simulink model "SimulationANTSMC"  (R2020b)
(part 1 of 18)
settings: Solver=ode3  StartTime=0.0  StopTime=100  FixedStep=0.001  RelTol=1e-6  EnableMultiTasking=on
model workspace (MAT data in the model file):
  time = 1
values from neighbouring files (symbols this model uses):
  beta = 2*x(3)/(1+x(3))    [GA_init.m]
  epstar = x(9)    [GA_init.m]
  g0 = x(5)    [GA_init.m]
  g1 = x(6)    [GA_init.m]
  g2 = x(7)    [GA_init.m]
  g3 = x(8)    [GA_init.m]
  gamma = x(3)    [GA_init.m]
  kappa = x(11)    [GA_init.m]
  landa = x(1)    [GA_init.m]
  nu = x(2)    [GA_init.m]
  vu = x(4)    [GA_init.m]

== system SimulationANTSMC ==
  Constant : Constant  Value=[0.00000000001*ones(6,1);zeros(6,1)]
  Control signal : Scope
  Disturbance : Scope
  Joint Trajectory : Subsystem
  Psi : Scope
  S : Scope
  Subsystem : Subsystem
  To Workspace : ToWorkspace  VariableName=error  SampleTime=-1
  To Workspace1 : ToWorkspace  VariableName=control_signal  SampleTime=-1
  Uas : Scope
  error : Scope
  thetadot : Scope
  track : Scope  NumInputPorts=2
  wires:
  Joint Trajectory/1(thetad) -> track/1, Subsystem/1(Xd)
  Subsystem/2(Error) -> error/1, To Workspace/1
  Subsystem/5(Control Signal) -> Control signal/1, To Workspace1/1
  Subsystem/1(theta) -> track/2
  Subsystem/3(thetadot) -> thetadot/1
  Subsystem/4(S) -> S/1
  Subsystem/6(Disturbance) -> Disturbance/1
  Constant/1 -> Subsystem/2(Initial)
  Subsystem/7(Us) -> Uas/1
  Subsystem/8(Psi1) -> Psi/1

== system SimulationANTSMC/Joint Trajectory ==
  Clock1 : Clock
  Mux : Mux  Inputs=6
  Mux1 : Mux  Commented=on  Inputs=6
  Sine Wave Function : Sin  TimeSource=Use external signal  Frequency=0.1*2*pi  SampleTime=0
  Sine Wave Function1 : Sin  TimeSource=Use external signal  Frequency=0.1*2*pi  SampleTime=0
  Sine Wave Function2 : Sin  TimeSource=Use external signal  Frequency=0.1*2*pi  SampleTime=0
  Sine Wave Function3 : Sin  TimeSource=Use external signal  Amplitude=-1  Frequency=0.1*2*pi  SampleTime=0
  Sine Wave Function4 : Sin  TimeSource=Use external signal  Amplitude=-1  Frequency=0.1*2*pi  SampleTime=0
  Sine Wave Function5 : Sin  TimeSource=Use external signal  Amplitude=-1  Frequency=0.1*2*pi  SampleTime=0
  Step : Step  Commented=on  Time=0  After=-5  SampleTime=0
  Step1 : Step  Commented=on  Time=0  After=-5  SampleTime=0
  Step2 : Step  Commented=on  Time=0  After=-1  SampleTime=0
  Step3 : Step  Commented=on  Time=0  After=5  SampleTime=0
  Step4 : Step  Commented=on  Time=0  After=5  SampleTime=0
  Step5 : Step  Commented=on  Time=0  After=5  SampleTime=0
  thetad : Outport
  wires:
  Clock1/1 -> Sine Wave Function5/1, Sine Wave Function4/1, Sine Wave Function1/1, Sine Wave Function/1, Sine Wave Function2/1, Sine Wave Function3/1
  Step3/1 -> Mux1/4
  Step4/1 -> Mux1/5
  Step5/1 -> Mux1/6
  Step2/1 -> Mux1/1
  Step1/1 -> Mux1/2
  Step/1 -> Mux1/3
  Mux/1 -> thetad/1
  Sine Wave Function5/1 -> Mux/1
  Sine Wave Function4/1 -> Mux/2
  Sine Wave Function3/1 -> Mux/3
  Sine Wave Function2/1 -> Mux/4
  Sine Wave Function1/1 -> Mux/5
  Sine Wave Function/1 -> Mux/6

== system SimulationANTSMC/Subsystem ==
  Xd : Inport
  Initial : Inport  Port=2
  Clock : Clock
  Constant1 : Constant  Value=landa
  Derivative{,1..3} (4 alike) : Derivative
  Design Parameters : Constant  Value=[g0,g1,g2,g3,gamma,beta]'
  Integrator : Integrator  InitialConditionSource=external  InitialCondition=[1*ones(6,1);ones(6,1)]  UpperSaturationLimit=10000  LowerSaturationLimit=-10000  AbsoluteTolerance=-1  ZeroCross=off
  Integrator1 : Integrator  InitialCondition=[0*ones(6,1)]  UpperSaturationLimit=1000  LowerSaturationLimit=-1000  AbsoluteTolerance=-1
  Mux : Mux  Inputs=6
  S manifold : MATLAB Function  TreatAsAtomicUnit=on
  Signal Specification{,1..3} (4 alike) : SignalSpecification  Dimensions=6
  Sum : Sum  Inputs=-|+
  Sum1 : Sum  Inputs=+|+
  System Dynamics : MATLAB Function  TreatAsAtomicUnit=on
  Theta : Subsystem
  To Workspace2 : ToWorkspace  VariableName=time  SampleTime=-1
  U : MATLAB Function  TreatAsAtomicUnit=on
  Uas : Subsystem
  Ueq : MATLAB Function  TreatAsAtomicUnit=on
  theta : Outport
  Error : Outport  Port=2
  thetadot : Outport  Port=3
  S : Outport  Port=4
  Control Signal : Outport  Port=5
  Disturbance : Outport  Port=6
  Us : Outport  Port=7
  Psi1 : Outport  Port=8
  wires:
  Sum1/1 -> Integrator1/1  "S"
  Constant1/1 -> Ueq/5(landa)
  Signal Specification1/1 -> Ueq/9(thetadot), U/4(thetadot), System Dynamics/2(thetadot)
  Clock/1 -> System Dynamics/4(t), To Workspace2/1
  System Dynamics/2(y) -> Integrator/1
  Design Parameters/1 -> S manifold/1(despar), Ueq/4(despar)
  Integrator/1 -> Theta/1(In1)
  Derivative/1 -> Ueq/7(edot), Derivative3/1, S manifold/3(edot)
  Theta/2(thetadot) -> Signal Specification1/1, thetadot/1
  Theta/1(theta) -> Signal Specification/1
  Derivative2/1 -> Ueq/1(xddd)
  Derivative1/1 -> Derivative2/1
  Sum/1 -> Ueq/3(e), Error/1, S manifold/2(e), Derivative/1  "Error"
  Ueq/1(y) -> Signal Specification2/1
  Signal Specification/1 -> theta/1, Sum/2, Ueq/8(theta), U/3(theta), System Dynamics/3(theta)
  Mux/1 -> Sum1/1, Ueq/6(part)
  Xd/1 -> Derivative1/1, Sum/1
  System Dynamics/1(disturbance) -> Disturbance/1
  S manifold/5(z5) -> Mux/5
  S manifold/1(z1) -> Mux/1
  S manifold/3(z3) -> Mux/3
  S manifold/4(z4) -> Mux/4
  S manifold/6(z6) -> Mux/6
  S manifold/2(z2) -> Mux/2
  Signal Specification2/1 -> U/1(Ueq)
  U/1(u) -> Control Signal/1, System Dynamics/1(u)
  Initial/1 -> Integrator/2
  Uas/1(Uas) -> U/2(Uas), Us/1
  Uas/2(Psi) -> Psi1/1
  Derivative3/1 -> Sum1/2
  Integrator1/1 -> Signal Specification3/1, Ueq/2(S)
  Signal Specification3/1 -> Uas/1(S), S/1

== system SimulationANTSMC/Subsystem/Theta ==
  In1 : Inport
  Bus Creator2 : BusCreator  Commented=on  Inputs=6
  Bus Creator3 : BusCreator  Commented=on  Inputs=6
  Subsystem : Subsystem  Commented=on
  Subsystem1 : Subsystem  Commented=on
  Subsystem2 : Subsystem  Commented=on
  Subsystem3 : Subsystem  Commented=on
  Subsystem4 : Subsystem  Commented=on
  Subsystem5 : Subsystem  Commented=on
  Subsystem6 : Subsystem  Commented=on
  Terminator : Terminator
  Theta : Subsystem
  theta : Outport
  thetadot : Outport  Port=2
  wires:
  Subsystem/3(Out3) -> Subsystem3/1(In1)  "theta3"
  Subsystem/6(Out6) -> Subsystem6/1(In1)  "theta6"
  Subsystem/4(Out4) -> Subsystem4/1(In1)  "theta4"
  Subsystem/11(Out11) -> Bus Creator3/5
  Subsystem/1(Out1) -> Subsystem1/1(In1)  "theta1"
  Subsystem/9(Out9) -> Bus Creator3/3
  Subsystem/12(Out12) -> Bus Creator3/6
  Subsystem/5(Out5) -> Subsystem5/1(In1)  "theta5"
  Subsystem/10(Out10) -> Bus Creator3/4
  Subsystem/8(Out8) -> Bus Creator3/2
  Subsystem/2(Out2) -> Subsystem2/1(In1)  "theta2"
  Subsystem/7(Out7) -> Bus Creator3/1
  Subsystem2/1(Out1) -> Bus Creator2/2
  Subsystem1/1(Out1) -> Bus Creator2/1
  Subsystem6/1(Out1) -> Bus Creator2/6
  Subsystem3/1(Out1) -> Bus Creator2/3
  Subsystem4/1(Out1) -> Bus Creator2/4
  Subsystem5/1(Out1) -> Bus Creator2/5
  In1/1 -> Theta/1(In1)
  Theta/1(Theta Degree) -> Terminator/1
  Theta/2(thetadot) -> thetadot/1
  Theta/3(Theta Radian) -> theta/1

== system SimulationANTSMC/Subsystem/Uas ==
  S : Inport
  Add2 : Sum
  Constant1 : Constant  Value=epstar
  Constant2 : Constant  Value=kappa
  Constant3 : Constant  Value=nu
  Constant4 : Constant  Value=vu
  Integrator2 : Integrator
  MATLAB Function : MATLAB Function  TreatAsAtomicUnit=on
  MATLAB Function1 : MATLAB Function  TreatAsAtomicUnit=on
  Product : Product
  Signal Specification : SignalSpecification  Dimensions=6
  Uas : Outport
  Psi : Outport  Port=2
  wires:
  Integrator2/1 -> Add2/2, Psi/1  "Psi"
  Add2/1 -> Product/2  "S"
  Constant2/1 -> MATLAB Function1/2(kappa)
  Constant3/1 -> Add2/1
  Product/1 -> Uas/1
  Constant1/1 -> MATLAB Function/2(epstar)
  Constant4/1 -> MATLAB Function1/3(vu)
  MATLAB Function/1(sat) -> Product/1
  MATLAB Function1/1(psi_dot) -> Signal Specification/1
  S/1 -> MATLAB Function/1(s), MATLAB Function1/1(s)
  Signal Specification/1 -> Integrator2/1

== system SimulationANTSMC/Subsystem/Theta/Subsystem ==
  In1 : Inport
  Demux3 : Demux  Outputs=12
  Out1 : Outport
  Out2 : Outport  Port=2
  Out3 : Outport  Port=3
  Out4 : Outport  Port=4
  Out5 : Outport  Port=5
  Out6 : Outport  Port=6
  Out7 : Outport  Port=7
  Out8 : Outport  Port=8
  Out9 : Outport  Port=9
  Out10 : Outport  Port=10
  Out11 : Outport  Port=11
  Out12 : Outport  Port=12
  wires:
  Demux3/1 -> Out1/1
  Demux3/9 -> Out9/1
  Demux3/10 -> Out10/1
  Demux3/7 -> Out7/1
  In1/1 -> Demux3/1
  Demux3/8 -> Out8/1
  Demux3/11 -> Out11/1
  Demux3/5 -> Out5/1
  Demux3/3 -> Out3/1
  Demux3/2 -> Out2/1
  Demux3/4 -> Out4/1
  Demux3/6 -> Out6/1
  Demux3/12 -> Out12/1

== system SimulationANTSMC/Subsystem/Theta/Subsystem1 ==
  In1 : Inport
  Constant2 : Constant  Value=360
  Gain : Gain  Gain=pi/180
  Math Function : Math  Operator=rem  SignedPower=on
  Out1 : Outport
  wires:
  Math Function/1 -> Out1/1
  In1/1 -> Gain/1
  Constant2/1 -> Math Function/2
  Gain/1 -> Math Function/1

== system SimulationANTSMC/Subsystem/Theta/Subsystem2 ==
  In1 : Inport
  Constant2 : Constant  Value=360
  Gain : Gain  Gain=pi/180
  Math Function : Math  Operator=rem  SignedPower=on
  Out1 : Outport
  wires:
  Math Function/1 -> Out1/1
  In1/1 -> Gain/1
  Constant2/1 -> Math Function/2
  Gain/1 -> Math Function/1

== system SimulationANTSMC/Subsystem/Theta/Subsystem3 ==
  In1 : Inport
  Constant2 : Constant  Value=360
  Gain : Gain  Gain=pi/180
  Math Function : Math  Operator=rem  SignedPower=on
  Out1 : Outport
  wires:
  Math Function/1 -> Out1/1
  In1/1 -> Gain/1
  Constant2/1 -> Math Function/2
  Gain/1 -> Math Function/1

== system SimulationANTSMC/Subsystem/Theta/Subsystem4 ==
  In1 : Inport
  Constant2 : Constant  Value=360
  Gain : Gain  Gain=pi/180
  Math Function : Math  Operator=rem  SignedPower=on
  Out1 : Outport
  wires:
  Math Function/1 -> Out1/1
  In1/1 -> Gain/1
  Constant2/1 -> Math Function/2
  Gain/1 -> Math Function/1
(part 1 of 6)
settings Model: Creator=CAST ta 1400  LastModifiedBy=Hirsa
settings DataIOCC: ReturnWorkspaceOutputs=off
settings OptimizationCC: LifeSpan=inf
settings DebuggingCC: SFUnexpectedBacktrackingDiag=warning  SFNoUnconditionalDefaultTransitionDiag=warning  ArithmeticOperatorsInVariantConditions=warning
settings SFSimCC: SimUseLocalCustomCode=off  CustomCodeUndefinedFunction=UseInterfaceOnly
settings RTWCC: RTWUseLocalCustomCode=off
settings CodeAppCC: StateflowObjectComments=on
settings GRTTargetCC: TargetLangStandard=C89/C90 (ANSI)
settings ConfigComp: CovMetricSettings=dw  CovSaveCumulativeToWorkspaceVar=on  CovSaveSingleToWorkspaceVar=on  CovExternalEMLEnable=off

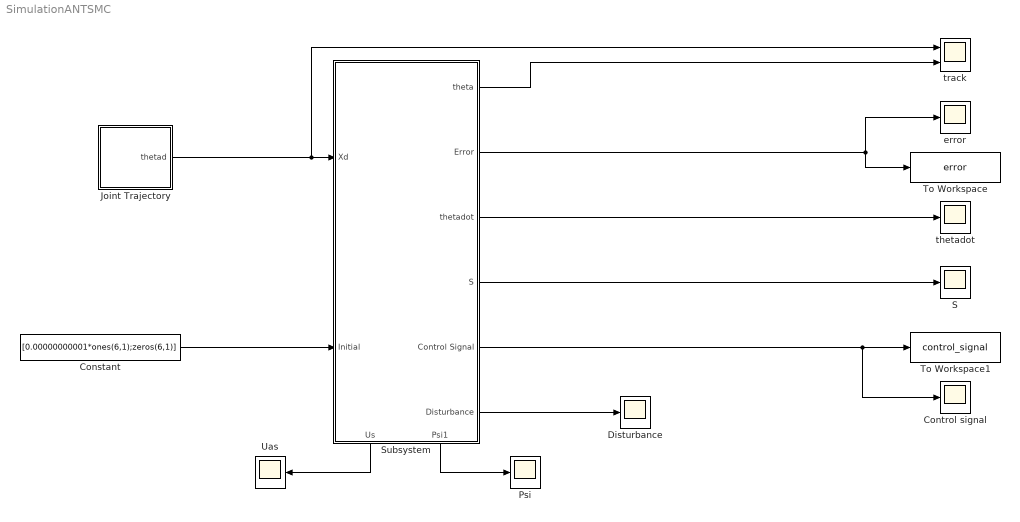
== system SimulationANTSMC ==
  Constant : Constant  Value=[0.00000000001*ones(6,1);zeros(6,1)]
  Control signal : Scope
  Disturbance : Scope
  Joint Trajectory : Subsystem
  Psi : Scope
  S : Scope
  Subsystem : Subsystem
      settings: PortSchema="{\"entries\":[{\"content\":{\"sides\":[{\"content\":{\"connectorIds\":[\"In1\",\"In2\"]},\"type\":\"ConnectorPlacement.EquallySpacedRectSide\",\"uuid\":\"6a081601-8c1c-4b92-8876-618e6a79f348\"},{\"content\":{\"connectorIds\":[\"Out1\",\"Out2\",\"Out3\",\"Out4\",\"Out5\",\"Out6\"],\"side\":\"RIGHT\"},\"type\":\"ConnectorPlacement.EquallySpacedRectSide\",\"uuid\":\"d972793b-0164-4612-badd-e3b053e392fc\"},{\"content\":{\"connectorIds\":[],\"side\":\"TOP\"},\"type\":\"ConnectorPlacement.EquallySpacedRectSide\",\"uuid\":\"780efbe4-9119-4fa0-8e03-d919fd60940e\"},{\"content\":{\"connectorIds\":[\"Out7\",\"Out8\"],\"side\":\"BOTTOM\"},\"type\":\"ConnectorPlacement.EquallySpacedRectSide\",\"uuid\":\"2e229f1a-e48e-496e-b525-7ed2e3990976\"},{\"content\":{\"connectorIds\":[],\"side\":\"HIDDEN\"},\"type\":\"ConnectorPlacement.EquallySpacedRectSide\",\"uuid\":\"e6c47cfa-e173-45ed-863d-94438e578280\"}]},\"type\":\"ConnectorPlacement.EquallySpacedConnector\",\"uuid\":\"71e70820-15e2-4153-83ec-01219cd454a2\"}],\"packageUris\":[\"http://schema.mathworks.com/mf0/Connector/R2020b\"],\"version\":\"1.0\"}"
  To Workspace : ToWorkspace  VariableName=error  SampleTime=-1
  To Workspace1 : ToWorkspace  VariableName=control_signal  SampleTime=-1
  Uas : Scope
  error : Scope
  thetadot : Scope
  track : Scope  NumInputPorts=2
  wires:
  Joint Trajectory/1(thetad) -> track/1, Subsystem/1(Xd)
  Subsystem/2(Error) -> error/1, To Workspace/1
  Subsystem/5(Control Signal) -> Control signal/1, To Workspace1/1
  Subsystem/1(theta) -> track/2
  Subsystem/3(thetadot) -> thetadot/1
  Subsystem/4(S) -> S/1
  Subsystem/6(Disturbance) -> Disturbance/1
  Constant/1 -> Subsystem/2(Initial)
  Subsystem/7(Us) -> Uas/1
  Subsystem/8(Psi1) -> Psi/1

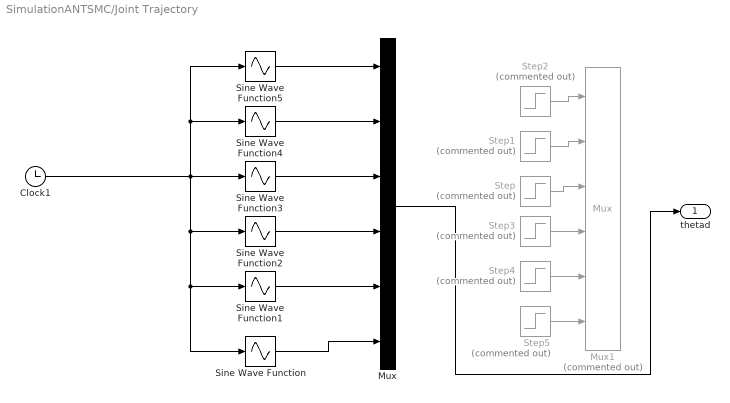
== system SimulationANTSMC/Joint Trajectory ==
  Clock1 : Clock
  Mux : Mux  Inputs=6
  Mux1 : Mux  Commented=on  Inputs=6
  Sine Wave Function : Sin  TimeSource=Use external signal  Frequency=0.1*2*pi  SampleTime=0
  Sine Wave Function1 : Sin  TimeSource=Use external signal  Frequency=0.1*2*pi  SampleTime=0
  Sine Wave Function2 : Sin  TimeSource=Use external signal  Frequency=0.1*2*pi  SampleTime=0
  Sine Wave Function3 : Sin  TimeSource=Use external signal  Amplitude=-1  Frequency=0.1*2*pi  SampleTime=0
  Sine Wave Function4 : Sin  TimeSource=Use external signal  Amplitude=-1  Frequency=0.1*2*pi  SampleTime=0
  Sine Wave Function5 : Sin  TimeSource=Use external signal  Amplitude=-1  Frequency=0.1*2*pi  SampleTime=0
  Step : Step  Commented=on  Time=0  After=-5  SampleTime=0
  Step1 : Step  Commented=on  Time=0  After=-5  SampleTime=0
  Step2 : Step  Commented=on  Time=0  After=-1  SampleTime=0
  Step3 : Step  Commented=on  Time=0  After=5  SampleTime=0
  Step4 : Step  Commented=on  Time=0  After=5  SampleTime=0
  Step5 : Step  Commented=on  Time=0  After=5  SampleTime=0
  thetad : Outport
  wires:
  Clock1/1 -> Sine Wave Function5/1, Sine Wave Function4/1, Sine Wave Function1/1, Sine Wave Function/1, Sine Wave Function2/1, Sine Wave Function3/1
  Step3/1 -> Mux1/4
  Step4/1 -> Mux1/5
  Step5/1 -> Mux1/6
  Step2/1 -> Mux1/1
  Step1/1 -> Mux1/2
  Step/1 -> Mux1/3
  Mux/1 -> thetad/1
  Sine Wave Function5/1 -> Mux/1
  Sine Wave Function4/1 -> Mux/2
  Sine Wave Function3/1 -> Mux/3
  Sine Wave Function2/1 -> Mux/4
  Sine Wave Function1/1 -> Mux/5
  Sine Wave Function/1 -> Mux/6

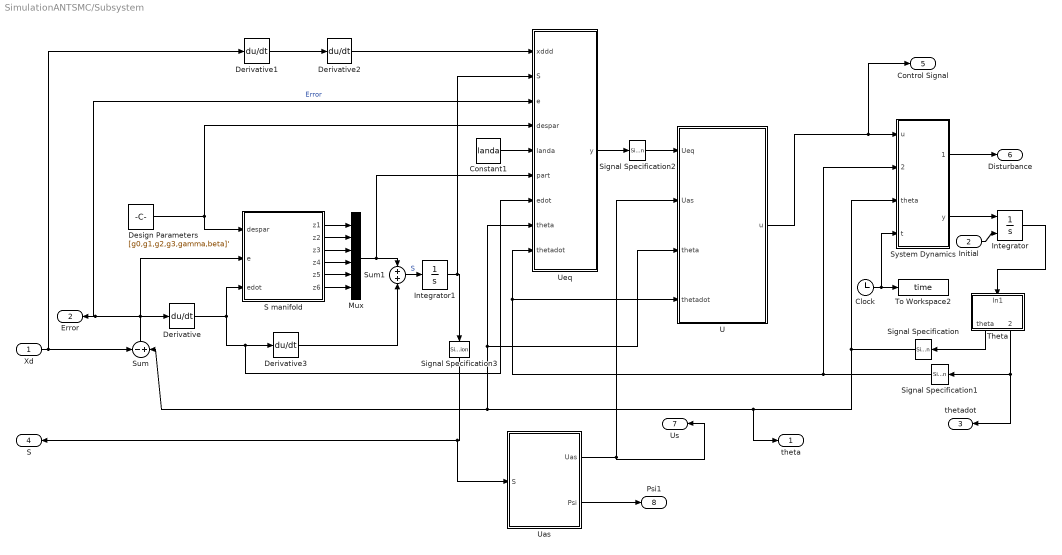
== system SimulationANTSMC/Subsystem ==
  Xd : Inport
  Initial : Inport  Port=2
  Clock : Clock
  Constant1 : Constant  Value=landa
  Derivative{,1..3} (4 alike) : Derivative
  Design Parameters : Constant  Value=[g0,g1,g2,g3,gamma,beta]'
  Integrator : Integrator  InitialConditionSource=external  InitialCondition=[1*ones(6,1);ones(6,1)]  UpperSaturationLimit=10000  LowerSaturationLimit=-10000  AbsoluteTolerance=-1  ZeroCross=off
  Integrator1 : Integrator  InitialCondition=[0*ones(6,1)]  UpperSaturationLimit=1000  LowerSaturationLimit=-1000  AbsoluteTolerance=-1
  Mux : Mux  Inputs=6
  S manifold : MATLAB Function  TreatAsAtomicUnit=on
  Signal Specification{,1..3} (4 alike) : SignalSpecification  Dimensions=6
  Sum : Sum  Inputs=-|+
  Sum1 : Sum  Inputs=+|+
  System Dynamics : MATLAB Function  TreatAsAtomicUnit=on
  Theta : Subsystem
  To Workspace2 : ToWorkspace  VariableName=time  SampleTime=-1
  U : MATLAB Function  TreatAsAtomicUnit=on
  Uas : Subsystem
  Ueq : MATLAB Function  TreatAsAtomicUnit=on
  theta : Outport
  Error : Outport  Port=2
  thetadot : Outport  Port=3
  S : Outport  Port=4
  Control Signal : Outport  Port=5
  Disturbance : Outport  Port=6
  Us : Outport  Port=7
  Psi1 : Outport  Port=8
  wires:
  Sum1/1 -> Integrator1/1  "S"
  Constant1/1 -> Ueq/5(landa)
  Signal Specification1/1 -> Ueq/9(thetadot), U/4(thetadot), System Dynamics/2(thetadot)
  Clock/1 -> System Dynamics/4(t), To Workspace2/1
  System Dynamics/2(y) -> Integrator/1
  Design Parameters/1 -> S manifold/1(despar), Ueq/4(despar)
  Integrator/1 -> Theta/1(In1)
  Derivative/1 -> Ueq/7(edot), Derivative3/1, S manifold/3(edot)
  Theta/2(thetadot) -> Signal Specification1/1, thetadot/1
  Theta/1(theta) -> Signal Specification/1
  Derivative2/1 -> Ueq/1(xddd)
  Derivative1/1 -> Derivative2/1
  Sum/1 -> Ueq/3(e), Error/1, S manifold/2(e), Derivative/1  "Error"
  Ueq/1(y) -> Signal Specification2/1
  Signal Specification/1 -> theta/1, Sum/2, Ueq/8(theta), U/3(theta), System Dynamics/3(theta)
  Mux/1 -> Sum1/1, Ueq/6(part)
  Xd/1 -> Derivative1/1, Sum/1
  System Dynamics/1(disturbance) -> Disturbance/1
  S manifold/5(z5) -> Mux/5
  S manifold/1(z1) -> Mux/1
  S manifold/3(z3) -> Mux/3
  S manifold/4(z4) -> Mux/4
  S manifold/6(z6) -> Mux/6
  S manifold/2(z2) -> Mux/2
  Signal Specification2/1 -> U/1(Ueq)
  U/1(u) -> Control Signal/1, System Dynamics/1(u)
  Initial/1 -> Integrator/2
  Uas/1(Uas) -> U/2(Uas), Us/1
  Uas/2(Psi) -> Psi1/1
  Derivative3/1 -> Sum1/2
  Integrator1/1 -> Signal Specification3/1, Ueq/2(S)
  Signal Specification3/1 -> Uas/1(S), S/1

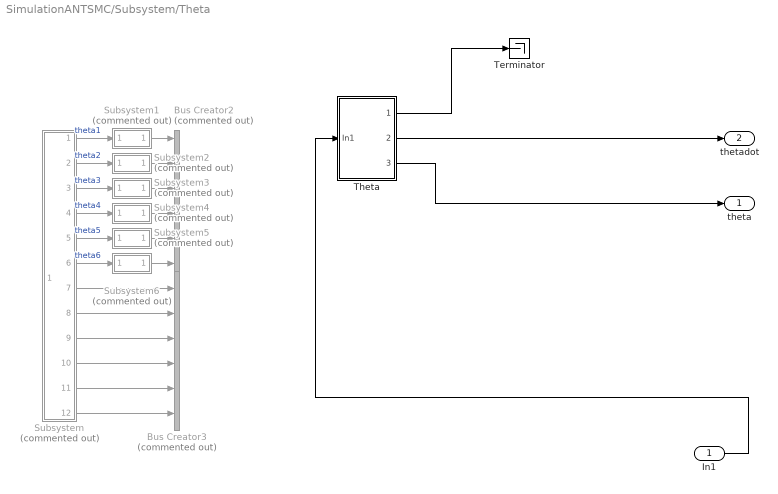
== system SimulationANTSMC/Subsystem/Theta ==
  In1 : Inport
  Bus Creator2 : BusCreator  Commented=on  Inputs=6
  Bus Creator3 : BusCreator  Commented=on  Inputs=6
  Subsystem : Subsystem  Commented=on
  Subsystem1 : Subsystem  Commented=on
  Subsystem2 : Subsystem  Commented=on
  Subsystem3 : Subsystem  Commented=on
  Subsystem4 : Subsystem  Commented=on
  Subsystem5 : Subsystem  Commented=on
  Subsystem6 : Subsystem  Commented=on
  Terminator : Terminator
  Theta : Subsystem
  theta : Outport
  thetadot : Outport  Port=2
  wires:
  Subsystem/3(Out3) -> Subsystem3/1(In1)  "theta3"
  Subsystem/6(Out6) -> Subsystem6/1(In1)  "theta6"
  Subsystem/4(Out4) -> Subsystem4/1(In1)  "theta4"
  Subsystem/11(Out11) -> Bus Creator3/5
  Subsystem/1(Out1) -> Subsystem1/1(In1)  "theta1"
  Subsystem/9(Out9) -> Bus Creator3/3
  Subsystem/12(Out12) -> Bus Creator3/6
  Subsystem/5(Out5) -> Subsystem5/1(In1)  "theta5"
  Subsystem/10(Out10) -> Bus Creator3/4
  Subsystem/8(Out8) -> Bus Creator3/2
  Subsystem/2(Out2) -> Subsystem2/1(In1)  "theta2"
  Subsystem/7(Out7) -> Bus Creator3/1
  Subsystem2/1(Out1) -> Bus Creator2/2
  Subsystem1/1(Out1) -> Bus Creator2/1
  Subsystem6/1(Out1) -> Bus Creator2/6
  Subsystem3/1(Out1) -> Bus Creator2/3
  Subsystem4/1(Out1) -> Bus Creator2/4
  Subsystem5/1(Out1) -> Bus Creator2/5
  In1/1 -> Theta/1(In1)
  Theta/1(Theta Degree) -> Terminator/1
  Theta/2(thetadot) -> thetadot/1
  Theta/3(Theta Radian) -> theta/1

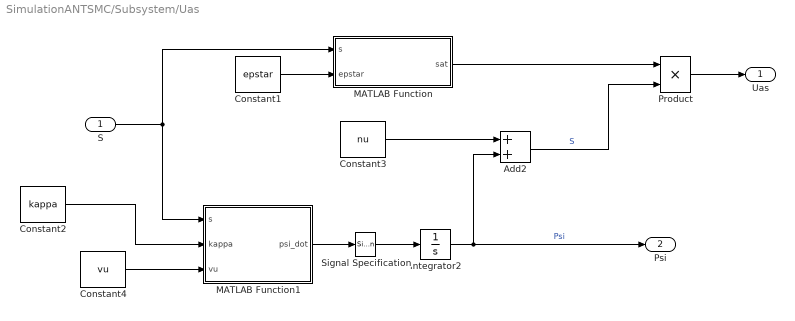
== system SimulationANTSMC/Subsystem/Uas ==
  S : Inport
  Add2 : Sum
  Constant1 : Constant  Value=epstar
  Constant2 : Constant  Value=kappa
  Constant3 : Constant  Value=nu
  Constant4 : Constant  Value=vu
  Integrator2 : Integrator
  MATLAB Function : MATLAB Function  TreatAsAtomicUnit=on
  MATLAB Function1 : MATLAB Function  TreatAsAtomicUnit=on
  Product : Product
  Signal Specification : SignalSpecification  Dimensions=6
  Uas : Outport
  Psi : Outport  Port=2
  wires:
  Integrator2/1 -> Add2/2, Psi/1  "Psi"
  Add2/1 -> Product/2  "S"
  Constant2/1 -> MATLAB Function1/2(kappa)
  Constant3/1 -> Add2/1
  Product/1 -> Uas/1
  Constant1/1 -> MATLAB Function/2(epstar)
  Constant4/1 -> MATLAB Function1/3(vu)
  MATLAB Function/1(sat) -> Product/1
  MATLAB Function1/1(psi_dot) -> Signal Specification/1
  S/1 -> MATLAB Function/1(s), MATLAB Function1/1(s)
  Signal Specification/1 -> Integrator2/1

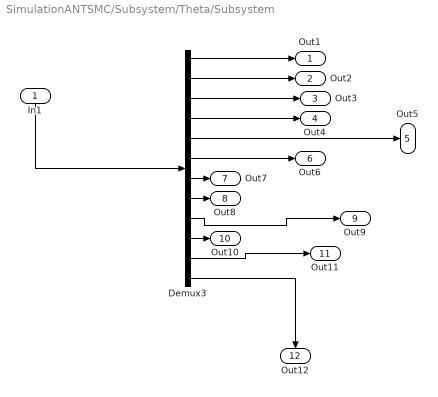
== system SimulationANTSMC/Subsystem/Theta/Subsystem ==
  In1 : Inport
  Demux3 : Demux  Outputs=12
  Out1 : Outport
  Out2 : Outport  Port=2
  Out3 : Outport  Port=3
  Out4 : Outport  Port=4
  Out5 : Outport  Port=5
  Out6 : Outport  Port=6
  Out7 : Outport  Port=7
  Out8 : Outport  Port=8
  Out9 : Outport  Port=9
  Out10 : Outport  Port=10
  Out11 : Outport  Port=11
  Out12 : Outport  Port=12
  wires:
  Demux3/1 -> Out1/1
  Demux3/9 -> Out9/1
  Demux3/10 -> Out10/1
  Demux3/7 -> Out7/1
  In1/1 -> Demux3/1
  Demux3/8 -> Out8/1
  Demux3/11 -> Out11/1
  Demux3/5 -> Out5/1
  Demux3/3 -> Out3/1
  Demux3/2 -> Out2/1
  Demux3/4 -> Out4/1
  Demux3/6 -> Out6/1
  Demux3/12 -> Out12/1

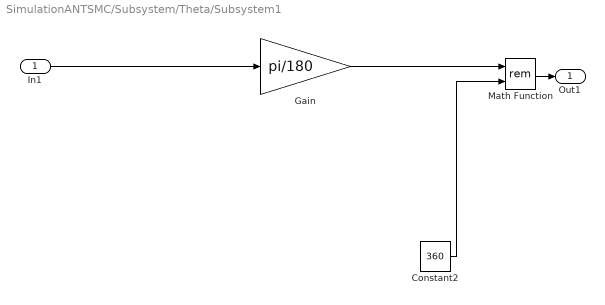
== system SimulationANTSMC/Subsystem/Theta/Subsystem1 ==
  In1 : Inport
  Constant2 : Constant  Value=360
  Gain : Gain  Gain=pi/180
  Math Function : Math  Operator=rem  SignedPower=on  SaturateOnIntegerOverflow=on
  Out1 : Outport
  wires:
  Math Function/1 -> Out1/1
  In1/1 -> Gain/1
  Constant2/1 -> Math Function/2
  Gain/1 -> Math Function/1

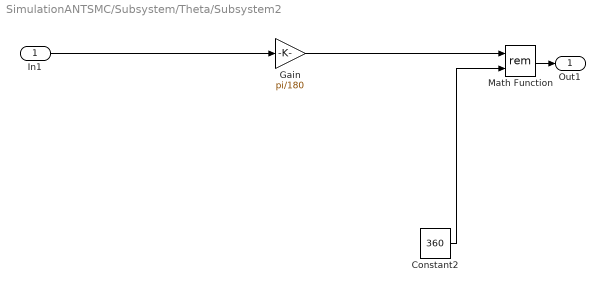
== system SimulationANTSMC/Subsystem/Theta/Subsystem2 ==
  In1 : Inport
  Constant2 : Constant  Value=360
  Gain : Gain  Gain=pi/180
  Math Function : Math  Operator=rem  SignedPower=on  SaturateOnIntegerOverflow=on
  Out1 : Outport
  wires:
  Math Function/1 -> Out1/1
  In1/1 -> Gain/1
  Constant2/1 -> Math Function/2
  Gain/1 -> Math Function/1

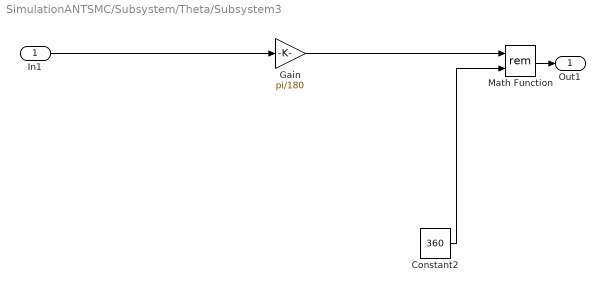
== system SimulationANTSMC/Subsystem/Theta/Subsystem3 ==
  In1 : Inport
  Constant2 : Constant  Value=360
  Gain : Gain  Gain=pi/180
  Math Function : Math  Operator=rem  SignedPower=on  SaturateOnIntegerOverflow=on
  Out1 : Outport
  wires:
  Math Function/1 -> Out1/1
  In1/1 -> Gain/1
  Constant2/1 -> Math Function/2
  Gain/1 -> Math Function/1

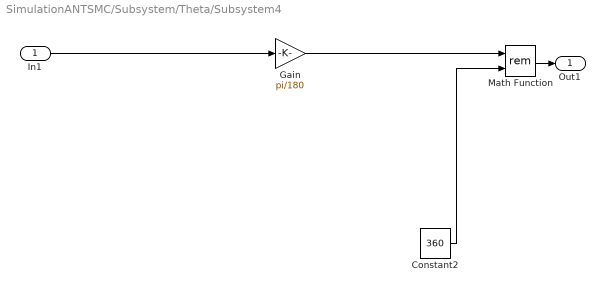
== system SimulationANTSMC/Subsystem/Theta/Subsystem4 ==
  In1 : Inport
  Constant2 : Constant  Value=360
  Gain : Gain  Gain=pi/180
  Math Function : Math  Operator=rem  SignedPower=on  SaturateOnIntegerOverflow=on
  Out1 : Outport
  wires:
  Math Function/1 -> Out1/1
  In1/1 -> Gain/1
  Constant2/1 -> Math Function/2
  Gain/1 -> Math Function/1

== system SimulationANTSMC/Subsystem/Theta/Subsystem5 ==
  In1 : Inport
  Constant2 : Constant  Value=360
  Gain : Gain  Gain=pi/180
  Math Function : Math  Operator=rem  SignedPower=on  SaturateOnIntegerOverflow=on
  Out1 : Outport
  wires:
  Math Function/1 -> Out1/1
  In1/1 -> Gain/1
  Constant2/1 -> Math Function/2
  Gain/1 -> Math Function/1

== system SimulationANTSMC/Subsystem/Theta/Subsystem6 ==
  In1 : Inport
  Constant2 : Constant  Value=360
  Gain : Gain  Gain=pi/180
  Math Function : Math  Operator=rem  SignedPower=on  SaturateOnIntegerOverflow=on
  Out1 : Outport
  wires:
  Math Function/1 -> Out1/1
  In1/1 -> Gain/1
  Constant2/1 -> Math Function/2
  Gain/1 -> Math Function/1

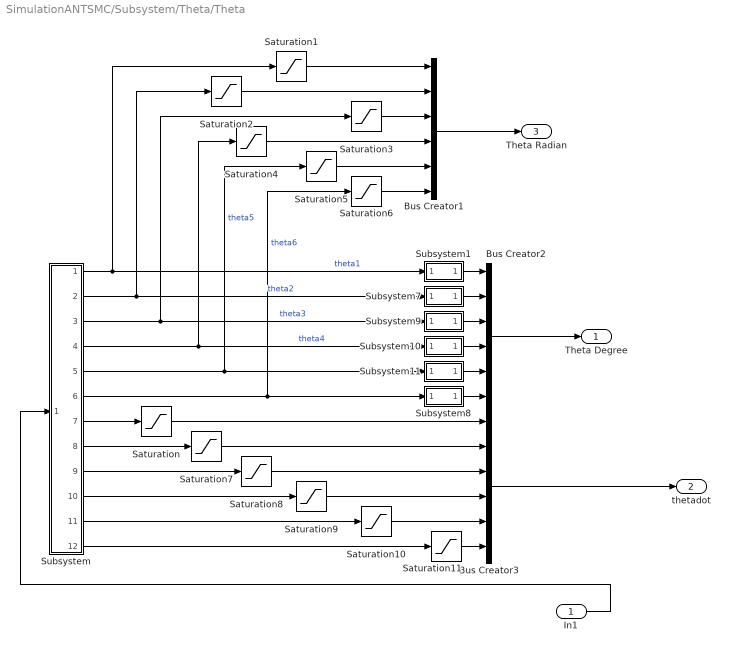
== system SimulationANTSMC/Subsystem/Theta/Theta ==
  In1 : Inport
  Bus Creator1 : BusCreator  Inputs=6
  Bus Creator2 : BusCreator  Inputs=6
  Bus Creator3 : BusCreator  Inputs=6
  Saturation : Saturate  UpperLimit=2.23  LowerLimit=-2.23
  Saturation1 : Saturate  UpperLimit=deg2rad(185)  LowerLimit=deg2rad(-185)
  Saturation10 : Saturate  UpperLimit=4.28  LowerLimit=-4.28
  Saturation11 : Saturate  UpperLimit=5.62  LowerLimit=-5.62
  Saturation2 : Saturate  UpperLimit=deg2rad(135)  LowerLimit=deg2rad(-135)
  Saturation3 : Saturate  UpperLimit=deg2rad(150)  LowerLimit=deg2rad(-150)
  Saturation4 : Saturate  UpperLimit=deg2rad(350)  LowerLimit=deg2rad(-350)
  Saturation5 : Saturate  UpperLimit=deg2rad(119)  LowerLimit=deg2rad(-119)
  Saturation6 : Saturate  UpperLimit=deg2rad(350)  LowerLimit=deg2rad(-350)
  Saturation7 : Saturate  UpperLimit=1.78  LowerLimit=-1.78
  Saturation8 : Saturate  UpperLimit=2.23  LowerLimit=-2.23
  Saturation9 : Saturate  UpperLimit=4.54  LowerLimit=-4.54
  Subsystem : Subsystem
  Subsystem1 : Subsystem
  Subsystem10 : Subsystem
  Subsystem11 : Subsystem
  Subsystem7 : Subsystem
  Subsystem8 : Subsystem
  Subsystem9 : Subsystem
  Theta Degree : Outport
  thetadot : Outport  Port=2
  Theta Radian : Outport  Port=3
  wires:
  In1/1 -> Subsystem/1(In1)
  Subsystem/11(Out11) -> Saturation10/1
  Subsystem/9(Out9) -> Saturation8/1
  Subsystem/12(Out12) -> Saturation11/1
  Subsystem/10(Out10) -> Saturation9/1
  Subsystem/8(Out8) -> Saturation7/1
  Subsystem/7(Out7) -> Saturation/1
  Subsystem7/1(Out1) -> Bus Creator2/2
  Subsystem1/1(Out1) -> Bus Creator2/1
  Subsystem8/1(Out1) -> Bus Creator2/6
  Subsystem9/1(Out1) -> Bus Creator2/3
  Subsystem10/1(Out1) -> Bus Creator2/4
  Subsystem11/1(Out1) -> Bus Creator2/5
  Subsystem/1(Out1) -> Saturation1/1, Subsystem1/1(In1)  "theta1"
  Subsystem/3(Out3) -> Subsystem9/1(In1), Saturation3/1  "theta3"
  Subsystem/4(Out4) -> Subsystem10/1(In1), Saturation4/1  "theta4"
  Subsystem/6(Out6) -> Subsystem8/1(In1), Saturation6/1  "theta6"
  Subsystem/5(Out5) -> Subsystem11/1(In1), Saturation5/1  "theta5"
  Subsystem/2(Out2) -> Subsystem7/1(In1), Saturation2/1  "theta2"
  Bus Creator1/1 -> Theta Radian/1
  Bus Creator2/1 -> Theta Degree/1
  Bus Creator3/1 -> thetadot/1
  Saturation1/1 -> Bus Creator1/1
  Saturation6/1 -> Bus Creator1/6
  Saturation5/1 -> Bus Creator1/5
  Saturation4/1 -> Bus Creator1/4
  Saturation3/1 -> Bus Creator1/3
  Saturation2/1 -> Bus Creator1/2
  Saturation11/1 -> Bus Creator3/6
  Saturation10/1 -> Bus Creator3/5
  Saturation9/1 -> Bus Creator3/4
  Saturation8/1 -> Bus Creator3/3
  Saturation7/1 -> Bus Creator3/2
  Saturation/1 -> Bus Creator3/1

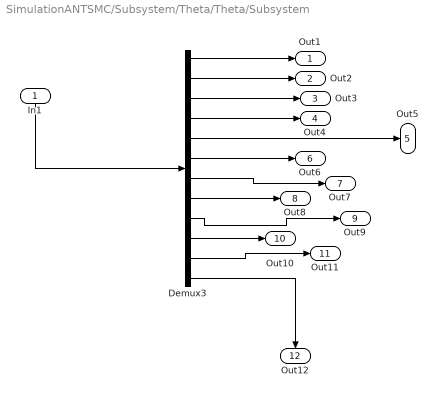
== system SimulationANTSMC/Subsystem/Theta/Theta/Subsystem ==
  In1 : Inport
  Demux3 : Demux  Outputs=12
  Out1 : Outport
  Out2 : Outport  Port=2
  Out3 : Outport  Port=3
  Out4 : Outport  Port=4
  Out5 : Outport  Port=5
  Out6 : Outport  Port=6
  Out7 : Outport  Port=7
  Out8 : Outport  Port=8
  Out9 : Outport  Port=9
  Out10 : Outport  Port=10
  Out11 : Outport  Port=11
  Out12 : Outport  Port=12
  wires:
  Demux3/1 -> Out1/1
  Demux3/9 -> Out9/1
  Demux3/10 -> Out10/1
  Demux3/7 -> Out7/1
  In1/1 -> Demux3/1
  Demux3/8 -> Out8/1
  Demux3/11 -> Out11/1
  Demux3/5 -> Out5/1
  Demux3/3 -> Out3/1
  Demux3/2 -> Out2/1
  Demux3/4 -> Out4/1
  Demux3/6 -> Out6/1
  Demux3/12 -> Out12/1

== system SimulationANTSMC/Subsystem/Theta/Theta/Subsystem1 ==
  In1 : Inport
  Constant2 : Constant  Value=360
  Gain : Gain  Gain=180/pi
  Math Function : Math  Operator=rem  SignedPower=on  SaturateOnIntegerOverflow=on
  Out1 : Outport
  wires:
  Math Function/1 -> Out1/1
  In1/1 -> Gain/1
  Constant2/1 -> Math Function/2
  Gain/1 -> Math Function/1

== system SimulationANTSMC/Subsystem/Theta/Theta/Subsystem10 ==
  In1 : Inport
  Constant2 : Constant  Value=360
  Gain : Gain  Gain=180/pi
  Math Function : Math  Operator=rem  SignedPower=on  SaturateOnIntegerOverflow=on
  Out1 : Outport
  wires:
  Math Function/1 -> Out1/1
  In1/1 -> Gain/1
  Constant2/1 -> Math Function/2
  Gain/1 -> Math Function/1

== system SimulationANTSMC/Subsystem/Theta/Theta/Subsystem11 ==
  In1 : Inport
  Constant2 : Constant  Value=360
  Gain : Gain  Gain=180/pi
  Math Function : Math  Operator=rem  SignedPower=on  SaturateOnIntegerOverflow=on
  Out1 : Outport
  wires:
  Math Function/1 -> Out1/1
  In1/1 -> Gain/1
  Constant2/1 -> Math Function/2
  Gain/1 -> Math Function/1

== system SimulationANTSMC/Subsystem/Theta/Theta/Subsystem7 ==
  In1 : Inport
  Constant2 : Constant  Value=360
  Gain : Gain  Gain=180/pi
  Math Function : Math  Operator=rem  SignedPower=on  SaturateOnIntegerOverflow=on
  Out1 : Outport
  wires:
  Math Function/1 -> Out1/1
  In1/1 -> Gain/1
  Constant2/1 -> Math Function/2
  Gain/1 -> Math Function/1

== system SimulationANTSMC/Subsystem/Theta/Theta/Subsystem8 ==
  In1 : Inport
  Constant2 : Constant  Value=360
  Gain : Gain  Gain=180/pi
  Math Function : Math  Operator=rem  SignedPower=on  SaturateOnIntegerOverflow=on
  Out1 : Outport
  wires:
  Math Function/1 -> Out1/1
  In1/1 -> Gain/1
  Constant2/1 -> Math Function/2
  Gain/1 -> Math Function/1

== system SimulationANTSMC/Subsystem/Theta/Theta/Subsystem9 ==
  In1 : Inport
  Constant2 : Constant  Value=360
  Gain : Gain  Gain=180/pi
  Math Function : Math  Operator=rem  SignedPower=on  SaturateOnIntegerOverflow=on
  Out1 : Outport
  wires:
  Math Function/1 -> Out1/1
  In1/1 -> Gain/1
  Constant2/1 -> Math Function/2
  Gain/1 -> Math Function/1
